simulink model "TANQUE_1_SIN_CONTROLslx"  (R2025b)
settings: Solver=ode45  StartTime=0.0  StopTime=200  RelTol=1e-3
settings Model: Creator=juerg

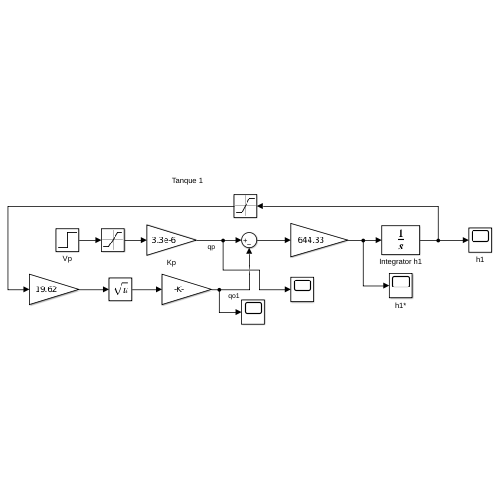
[thumbnail: Simulink's stored preview of the top-level diagram]
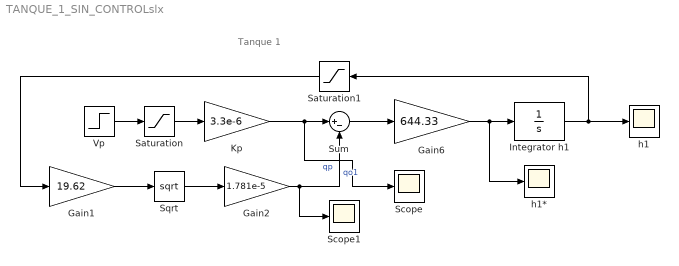
== system TANQUE_1_SIN_CONTROLslx ==
  note: Tanque 1
  Gain1 : Gain  Gain=19.62
  Gain2 : Gain  Gain=1.781e-5
  Gain6 : Gain  Gain=644.33
  Integrator h1 : Integrator
  Kp : Gain  Gain=3.3e-6
  Saturation : Saturate  UpperLimit=10  LowerLimit=0
  Saturation1 : Saturate  UpperLimit=Inf  LowerLimit=0
  Scope : Scope
      settings: ActiveDisplayYMinimum=-2.0624999999999997E-6  ActiveDisplayYMaximum=1.85625E-5  DataLoggingVariableName=ScopeData4
  Scope1 : Scope
      settings: ActiveDisplayYMinimum=-1  ActiveDisplayYMaximum=1  DataLoggingVariableName=ScopeData5
  Sqrt : Sqrt
  Sum : Sum  Inputs=|+-
  Vp : Step  After=10  SampleTime=0
  h1 : Scope
      settings: ActiveDisplayYMinimum=-0.021873045482770158  ActiveDisplayYMaximum=0.19685740934493146
  h1* : Scope
      settings: ActiveDisplayYMinimum=-0.0013392843750000022  ActiveDisplayYMaximum=0.012053559375  DataLoggingVariableName=ScopeData2
  wires:
  Vp/1 -> Saturation/1
  Gain1/1 -> Sqrt/1
  Sqrt/1 -> Gain2/1
  Kp/1 -> Scope/1, Sum/1  "qp"
  Gain2/1 -> Scope1/1, Sum/2  "qo1"
  Sum/1 -> Gain6/1
  Gain6/1 -> h1*/1, Integrator h1/1
  Integrator h1/1 -> h1/1, Saturation1/1
  Saturation/1 -> Kp/1
  Saturation1/1 -> Gain1/1
